simulink model "testemotor"  (R2023a)
settings: Solver=VariableStepAuto  StartTime=0.0  StopTime=10  RelTol=1e-3
values from neighbouring files (symbols this model uses):
  B = 0.3441    [datos_planta.m]
  J = 0.0112    [datos_planta.m]
  Ka = 0.2335    [datos_planta.m]
  Km = 0.147    [datos_planta.m]
  L = 0.52    [datos_planta.m]
  R = 1.6    [datos_planta.m]
libraries: ee_lib x1
settings Model: Creator=hiago.sodre  LastModifiedBy=hiago.sodre

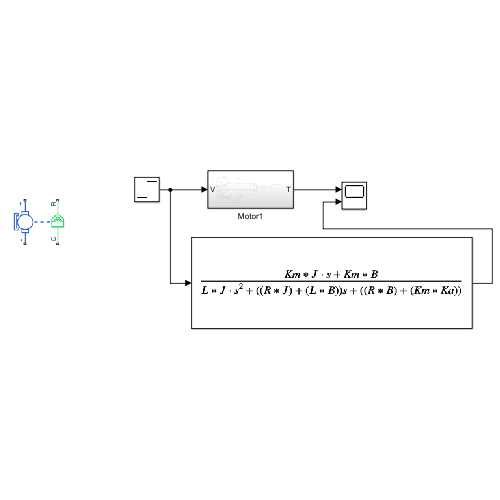
[thumbnail: Simulink's stored preview of the top-level diagram]
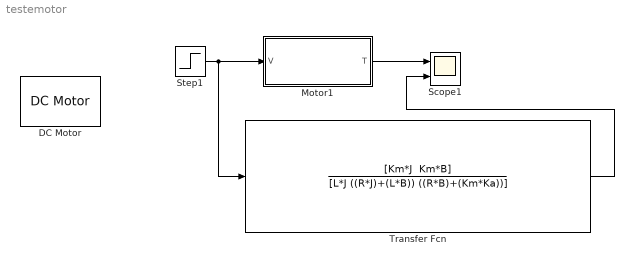
== system testemotor ==
  DC Motor : ee_lib/Electromechanical/Brushed Motors/DC Motor  field_option=ee.enum.field_option.pm  Rf=100 Ohm  Lf=1 H  Laf=0.15 H  If0=0 A  parameterization=ee.enum.dcparam_option.torque_speed  Ra=3.9 Ohm  La=12e-6 H  emf_or_torque=ee.enum.emf_or_torque.kv  Kv=0.072e-3 V/rpm  Ki=6.876e-4 N*m/A  T_stall=0.24e-3 N*m  w_max=19100 rpm  w_rated=15000 rpm  P_rated=0.08 W  V_rated=1.5 V  lam_param=ee.enum.lam_param.damping  i_noload=0 A  V_i_noload=1.5 V  J=0.01 cm^2*g  lam=0 N*m*s/rad  speed0=0 rpm  enable_fault_armature=simscape.enum.onoff.off  rev_faulted=1 / 3  G_faulted_armature=1e-5 S  fault_trigger_armature=ee.enum.faults.faultTrigger.temporal  t_fault_armature=1 s  max_permissible_current_armature=inf A  t_fail_on_current_armature=1 s  enable_fault_field=simscape.enum.onoff.off  G_faulted_field=1e-5 S  fault_trigger_field=ee.enum.faults.faultTrigger.temporal  t_fault_field=1 s  max_permissible_current_field=inf A  t_fail_on_current_field=1 s  fault_action=simscape.enum.assert.action.none  alpha=3.93e-3 1/K  Tmeas=25 degC  thermal_mass=100 J/K  initial_temperature=25 degC
  Motor1 : Subsystem
  Scope1 : Scope  NumInputPorts=2
  Step1 : Step  After=6  SampleTime=1
  Transfer Fcn : TransferFcn  Numerator="[Km*J  Km*B]"  Denominator=[L*J ((R*J)+(L*B)) ((R*B)+(Km*Ka))]
  wires:
  Motor1/1(T) -> Scope1/1
  Step1/1 -> Transfer Fcn/1, Motor1/1(V)
  Transfer Fcn/1 -> Scope1/2

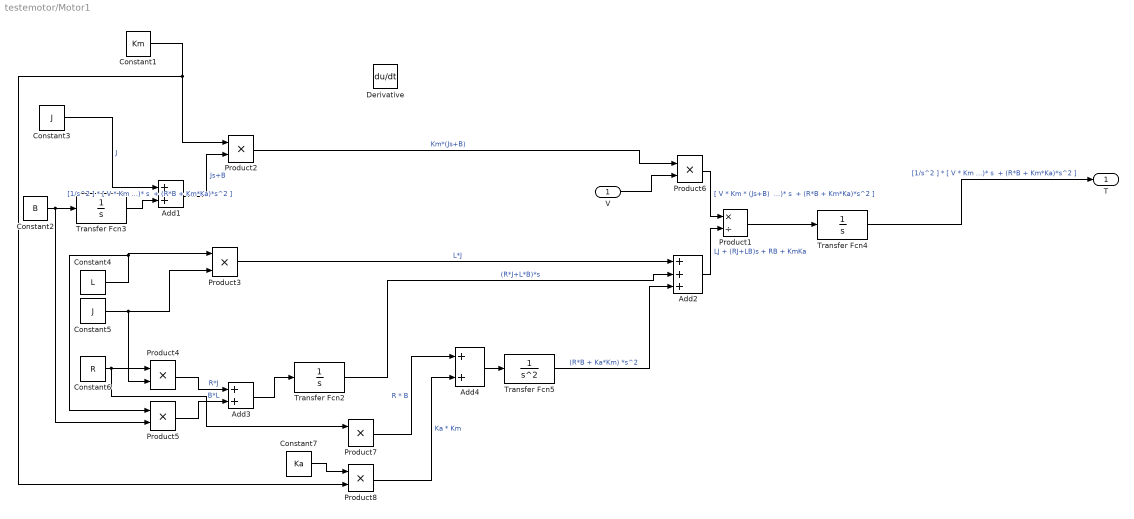
== system testemotor/Motor1 ==
  V : Inport
  Add1 : Sum
  Add2 : Sum  Inputs=+++
  Add3 : Sum
  Add4 : Sum
  Constant1 : Constant  Value=Km
  Constant2 : Constant  Value=B
  Constant3 : Constant  Value=J
  Constant4 : Constant  Value=L
  Constant5 : Constant  Value=J
  Constant6 : Constant  Value=R
  Constant7 : Constant  Value=Ka
  Derivative : Derivative
  Product1 : Product  Inputs=*/
  Product{2..8} (7 alike) : Product
  Transfer Fcn2 : TransferFcn  Denominator=[0 1 0]
  Transfer Fcn3 : TransferFcn  Denominator=[1 0]
  Transfer Fcn4 : TransferFcn  Denominator=[1 0]
  Transfer Fcn5 : TransferFcn  Denominator=[1 0 0]
  T : Outport
  wires:
  Add1/1 -> Product2/2  "Js+B"
  Product2/1 -> Product6/1  "Km*(Js+B)"
  Constant5/1 -> Product3/2, Product4/2
  Constant4/1 -> Product5/1, Product3/1
  Product4/1 -> Add3/1  "R*J"
  Product5/1 -> Add3/2  "B*L"
  Add2/1 -> Product1/2  "LJ + (RJ+LB)s + RB + KmKa"
  Add3/1 -> Transfer Fcn2/1
  Transfer Fcn2/1 -> Add2/2  "(R*J+L*B)*s"
  Constant6/1 -> Product7/1, Product4/1
  Product7/1 -> Add4/1  "R * B"
  Constant7/1 -> Product8/1
  Constant1/1 -> Product2/1, Product8/2
  Product8/1 -> Add4/2  "Ka * Km"
  Constant3/1 -> Add1/1  "J"
  Product3/1 -> Add2/1  "L*J"
  Transfer Fcn4/1 -> T/1  "[1/s^2 ] * [ V * Km * (Js+B)  /  L*J + (RJ+LB)* s  + (R*B + Km*Ka)*s^2 ]"
  V/1 -> Product6/2
  Product6/1 -> Product1/1  "[ V * Km * (Js+B)  /  L*J + (RJ+LB)* s  + (R*B + Km*Ka)*s^2 ]"
  Product1/1 -> Transfer Fcn4/1
  Add4/1 -> Transfer Fcn5/1
  Transfer Fcn5/1 -> Add2/3  "(R*B + Ka*Km) *s^2"
  Constant2/1 -> Product5/2, Transfer Fcn3/1
  Transfer Fcn3/1 -> Add1/2  "[1/s^2 ] * [ V * Km * (Js+B)  /  L*J + (RJ+LB)* s  + (R*B + Km*Ka)*s^2 ]"
